simulink model "damping"  (R2014a)
settings: Solver=ode45  StartTime=0.0  StopTime=10.0  RelTol=1e-3
settings Model: Creator=Grid  LastModifiedBy=Grid

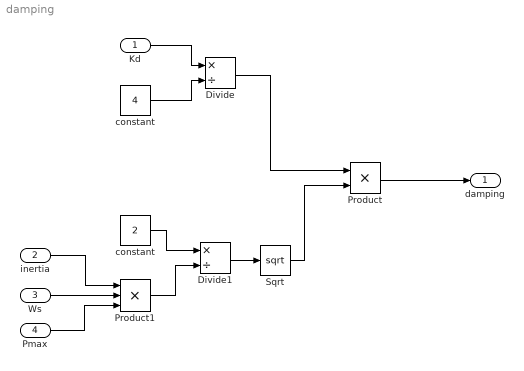
== system damping ==
  Kd : Inport  RequirementInfo={} %GIDa_4bc4385b_0099_4f67_b2c8_5e52b80bfdb4
  "inertia " : Inport  RequirementInfo={} %GIDa_5aa97e76_d8bf_4540_a945_5c6e3660522e  Port=2
  Ws : Inport  RequirementInfo={} %GIDa_4b89831b_fe31_4538_8d3d_4c8afd9c7bdb  Port=3
  Pmax : Inport  RequirementInfo={} %GIDa_0f3ffebd_5683_4346_b3dc_dd08a2a9df8a  Port=4
  Divide : Product  Inputs=*/
  Divide1 : Product  Inputs=*/
  Product : Product
  Product1 : Product  Inputs=3
  Sqrt : Sqrt  SaturateOnIntegerOverflow=on
  constant : Constant  Value=2  VectorParams1D=off
  "constant " : Constant  Value=4  VectorParams1D=off
  damping : Outport  RequirementInfo={'linktype_rmi_matlab' 'Diesel' '@736250.1' 'true' 'damping' '' } %GIDa_02eca54f_d355_4587_be72_9bd749126863
  wires:
  Kd/1 -> Divide/1
  "constant "/1 -> Divide/2
  Ws/1 -> Product1/2
  constant/1 -> Divide1/1
  "inertia "/1 -> Product1/1
  Pmax/1 -> Product1/3
  Product1/1 -> Divide1/2
  Divide1/1 -> Sqrt/1
  Sqrt/1 -> Product/2
  Divide/1 -> Product/1
  Product/1 -> damping/1
